simulink model "F_Control_of_2_Area"  (R2021b)
settings: Solver=VariableStepAuto  StartTime=0.0  StopTime=100.0  RelTol=1e-3  EnableMultiTasking=on
settings Model: Creator=user  LastModifiedBy=HP
settings SolverCC: AlgebraicLoopSolver=TrustRegion
settings DataIOCC: ReturnWorkspaceOutputs=off
settings OptimizationCC: LifeSpan=inf
settings DebuggingCC: SFUnexpectedBacktrackingDiag=warning  SFNoUnconditionalDefaultTransitionDiag=warning  SFMachineParentedDataDiag=warning  ArithmeticOperatorsInVariantConditions=warning
settings SFSimCC: SimUseLocalCustomCode=off  CustomCodeUndefinedFunction=UseInterfaceOnly
settings RTWCC: RTWUseLocalCustomCode=off
settings CodeAppCC: StateflowObjectComments=on
settings GRTTargetCC: TargetLangStandard=C89/C90 (ANSI)
settings ConfigComp: CovMetricSettings=dw  CovSaveCumulativeToWorkspaceVar=on  CovSaveSingleToWorkspaceVar=on  CovExternalEMLEnable=off

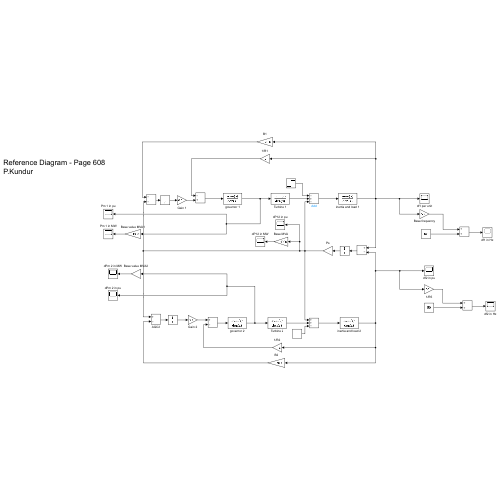
[thumbnail: Simulink's stored preview of the top-level diagram]
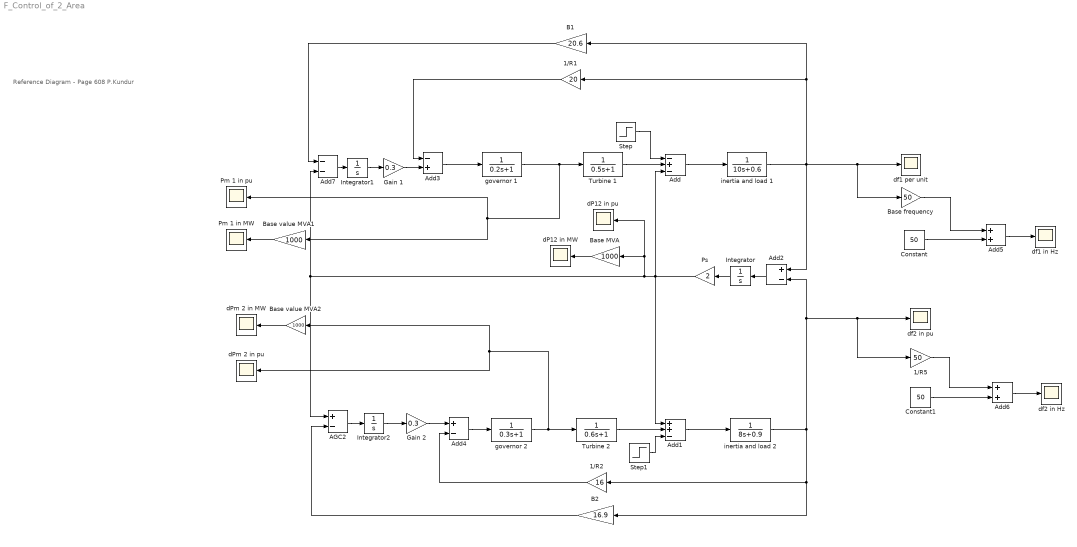
== system F_Control_of_2_Area ==
  note: Reference Diagram - Page 608 P.Kundur
  1/R1 : Gain  Gain=20
  1/R2 : Gain  Gain=16
  1/R5 : Gain  Gain=50
  AGC2 : Sum  Inputs=+-
  Add : Sum  Inputs=-+-
  Add1 : Sum  Inputs=++-
  Add2 : Sum  Inputs=+-
  Add3 : Sum  Inputs=-+
  Add4 : Sum  Inputs=+-
  Add5 : Sum
  Add6 : Sum
  Add7 : Sum  Inputs=--
  B1 : Gain  Gain=20.6
  B2 : Gain  Gain=16.9
  Base MVA : Gain  Gain=1000
  Base frequency : Gain  Gain=50
  Base value MVA1 : Gain  Gain=1000
  Base value MVA2 : Gain  Gain=1000
  Constant : Constant  Value=50
  Constant1 : Constant  Value=50
  Gain 1 : Gain  Gain=0.3
  Gain 2 : Gain  Gain=0.3
  Integrator : Integrator
  Integrator1 : Integrator
  Integrator2 : Integrator
  Pm 1 in MW : Scope
  Pm 1 in pu : Scope
  Ps : Gain  Gain=2
  Step : Step  Time=100  Before=0.1875  After=0.1875  SampleTime=0
  Step1 : Step  Time=100  Before=-0.05  After=0.05  SampleTime=0
  Turbine 1 : TransferFcn  Denominator=[0.5 1]
  Turbine 2 : TransferFcn  Denominator=[0.6 1]
  dP12 in MW : Scope
  dP12 in pu : Scope
  dPm 2 in MW : Scope
  dPm 2 in pu : Scope
  df1 in Hz : Scope
  df1 per unit : Scope
  df2 in Hz : Scope
  df2 in pu : Scope
  governor 1 : TransferFcn  Denominator=[0.2 1]
  governor 2 : TransferFcn  Denominator=[0.3 1]
  inertia and load 1 : TransferFcn  Denominator=[10 0.6]
  inertia and load 2 : TransferFcn  Denominator=[8 0.9]
  wires:
  Add/1 -> inertia and load 1/1
  Turbine 1/1 -> Add/2
  Add3/1 -> governor 1/1
  inertia and load 1/1 -> Add2/1, Base frequency/1, df1 per unit/1, B1/1, 1/R1/1
  Add1/1 -> inertia and load 2/1
  Turbine 2/1 -> Add1/2
  inertia and load 2/1 -> df2 in pu/1, 1/R5/1, Add2/2, 1/R2/1, B2/1
  governor 2/1 -> dPm 2 in pu/1, Base value MVA2/1, Turbine 2/1
  governor 1/1 -> Turbine 1/1, Pm 1 in pu/1, Base value MVA1/1
  Add2/1 -> Integrator/1
  Integrator/1 -> Ps/1
  Ps/1 -> Add/3, Base MVA/1, dP12 in pu/1, Add7/2, AGC2/1, Add1/1
  Step/1 -> Add/1
  1/R1/1 -> Add3/1
  Add4/1 -> governor 2/1
  Base frequency/1 -> Add5/1
  1/R5/1 -> Add6/1
  Constant/1 -> Add5/2
  Add5/1 -> df1 in Hz/1
  Constant1/1 -> Add6/2
  Add6/1 -> df2 in Hz/1
  Base value MVA1/1 -> Pm 1 in MW/1
  Base value MVA2/1 -> dPm 2 in MW/1
  Base MVA/1 -> dP12 in MW/1
  B1/1 -> Add7/1
  Add7/1 -> Integrator1/1
  B2/1 -> AGC2/2
  AGC2/1 -> Integrator2/1
  1/R2/1 -> Add4/2
  Integrator1/1 -> Gain 1/1
  Gain 1/1 -> Add3/2
  Integrator2/1 -> Gain 2/1
  Gain 2/1 -> Add4/1
  Step1/1 -> Add1/3
